simulink model "feedback_plant_with_simple_v2_PID"  (R2016a)
settings: Solver=FixedStepAuto  StartTime=0.0  StopTime=5580  MaxStep=0.1  RelTol=1e-3
undefined symbols (not defined in the file): sensors
libraries: slrtlib x10, simulink x3, xpcnilib x2
settings Model: ModifiedByFormat=The MathWorks Inc.  Creator=The MathWorks, Inc.  LastModifiedBy=The MathWorks Inc.
settings SolverCC: EnableConcurrentExecution=on
settings DataIOCC: LimitDataPoints=on  SaveFormat=Array
settings OptimizationCC: BlockReduction=off  DefaultParameterBehavior=Inlined  OptimizeBlockIOStorage=off  BufferReuse=off  GlobalBufferReuse=off  ExpressionFolding=off  ExpressionDepthLimit=2147483647  LocalBlockOutputs=off
settings DebuggingCC: UnderspecifiedInitializationDetection=Classic  MergeDetectMultiDrivingBlocksExec=none  SolverPrmCheckMsg=warning  FcnCallInpInsideContextMsg=EnableAllAsWarning  AllowSymbolicDim=off  StateNameClashWarn=warning
settings HardwareCC: ProdBitPerPointer=32  ProdLargestAtomicFloat=None  ProdWordSize=32  ProdLongLongMode=on  ProdHWDeviceType=Generic->32-bit x86 compatible
settings ModelReferenceCC: ModelReferenceNumInstancesAllowed=Single  ModelReferenceMinAlgLoopOccurrences=on  PropagateSignalLabelsOutOfModel=off
settings RTWCC: SystemTargetFile=slrt.tlc  TemplateMakefile=slrt_default_tmf  Description=Simulink Real-Time  RTWVerbose=off
settings ConfigComp: CovModelRefEnable=Off  CovSFcnEnable=off

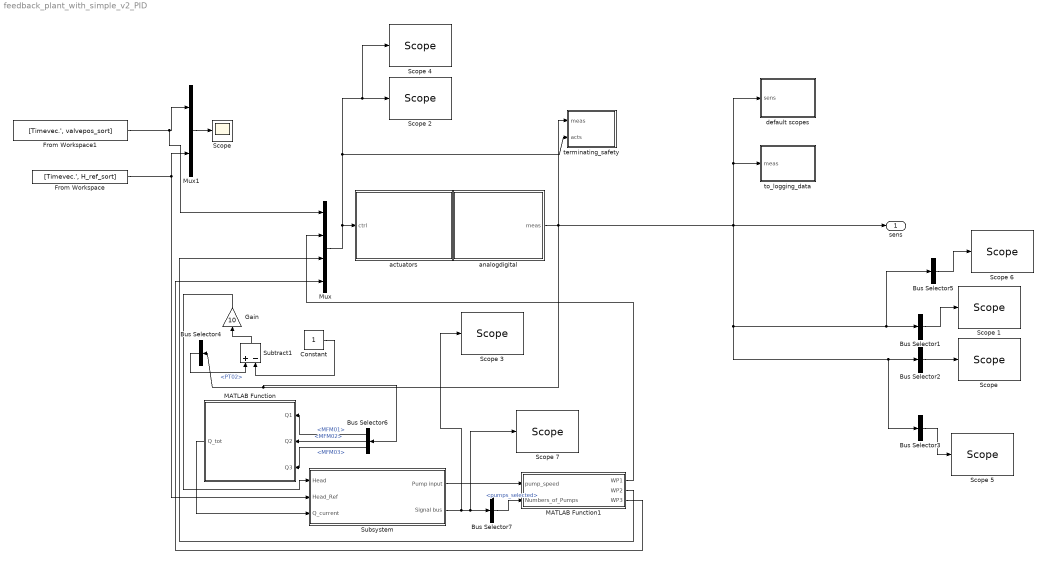
== system feedback_plant_with_simple_v2_PID ==
  Bus Selector1 : BusSelector  OutputSignals=CV01,DPT01,DPT02,DPT03,MFM01,MFM02,MFM03,PT02  OutputAsBus=on
  Bus Selector2 : BusSelector  OutputSignals=LMGV1,LMGV2,LMGV3,LMGC1,LMGC2,LMGC3,LMGP1,LMGP2,LMGP3  OutputAsBus=on
  Bus Selector3 : BusSelector  OutputSignals=WP01,WP02,WP03  OutputAsBus=on
  Bus Selector4 : BusSelector  OutputSignals=PT02
  Bus Selector5 : BusSelector  OutputSignals=PT02  OutputAsBus=on
  Bus Selector6 : BusSelector  OutputSignals=MFM01,MFM02,MFM03
  Bus Selector7 : BusSelector  OutputSignals=pumps_selected
  Constant : Constant
  From Workspace : FromWorkspace  VariableName=[Timevec.', H_ref_sort]  SampleTime=0  Interpolate=off  OutputAfterFinalValue=Holding final value
  From Workspace1 : FromWorkspace  VariableName=[Timevec.', valvepos_sort]  SampleTime=0  Interpolate=off  OutputAfterFinalValue=Holding final value
  Gain : Gain  Gain=10
  MATLAB Function : MATLAB Function  TreatAsAtomicUnit=on
  MATLAB Function1 : MATLAB Function  TreatAsAtomicUnit=on
  Mux : Mux
  Mux1 : Mux  Inputs=2
  Scope : Scope
  "Scope " : slrtlib/Displays and Logging/Scope   scopeno=9  scopetype=Target  autostart=on  viewmode=Numerical  formatstr='%15.6f'  grid=on  ylimits=[0,0]  nosamples=25  noprepostsamples=0  interleave=1  triggermode=FreeRun  triggersignal=1  trigsignalfromport=off  triggerlevel=0.0  triggerslope=Either  triggerscope=1  triggersample=0  filename=data.dat  mode=Lazy  writesize=512  autorestart=off  dynamicfilemode=off  maxwritefilesize=512*1024^2
  Scope 1 : slrtlib/Displays and Logging/Scope   scopeno=10  scopetype=Target  autostart=on  viewmode=Numerical  formatstr='%15.6f'  grid=on  ylimits=[0,0]  nosamples=25  noprepostsamples=0  interleave=1  triggermode=FreeRun  triggersignal=1  trigsignalfromport=off  triggerlevel=0.0  triggerslope=Either  triggerscope=1  triggersample=0  filename=data.dat  mode=Lazy  writesize=512  autorestart=off  dynamicfilemode=off  maxwritefilesize=512*1024^2
  Scope 2 : slrtlib/Displays and Logging/Scope   scopeno=2  scopetype=Host  autostart=on  viewmode=Graphical redraw  formatstr='%15.6f'  grid=on  ylimits=[0,0]  nosamples=250  noprepostsamples=0  interleave=1  triggermode=FreeRun  triggersignal=1  trigsignalfromport=off  triggerlevel=0.0  triggerslope=Either  triggerscope=1  triggersample=0  filename=data.dat  mode=Lazy  writesize=512  autorestart=off  dynamicfilemode=off  maxwritefilesize=512*1024^2
  Scope 3 : slrtlib/Displays and Logging/Scope   scopeno=3  scopetype=Host  autostart=on  viewmode=Graphical redraw  formatstr='%15.6f'  grid=on  ylimits=[0,0]  nosamples=250  noprepostsamples=0  interleave=1  triggermode=FreeRun  triggersignal=1  trigsignalfromport=off  triggerlevel=0.0  triggerslope=Either  triggerscope=1  triggersample=0  filename=data.dat  mode=Lazy  writesize=512  autorestart=off  dynamicfilemode=off  maxwritefilesize=512*1024^2
  Scope 4 : slrtlib/Displays and Logging/Scope   scopeno=8  scopetype=Target  autostart=on  viewmode=Numerical  formatstr='%15.6f'  grid=on  ylimits=[0,0]  nosamples=25  noprepostsamples=0  interleave=1  triggermode=FreeRun  triggersignal=1  trigsignalfromport=off  triggerlevel=0.0  triggerslope=Either  triggerscope=1  triggersample=0  filename=data.dat  mode=Lazy  writesize=512  autorestart=off  dynamicfilemode=off  maxwritefilesize=512*1024^2
  Scope 5 : slrtlib/Displays and Logging/Scope   scopeno=11  scopetype=Target  autostart=on  viewmode=Numerical  formatstr='%15.6f'  grid=on  ylimits=[0,0]  nosamples=25  noprepostsamples=0  interleave=1  triggermode=FreeRun  triggersignal=1  trigsignalfromport=off  triggerlevel=0.0  triggerslope=Either  triggerscope=1  triggersample=0  filename=data.dat  mode=Lazy  writesize=512  autorestart=off  dynamicfilemode=off  maxwritefilesize=512*1024^2
  Scope 6 : slrtlib/Displays and Logging/Scope   scopeno=4  scopetype=Target  autostart=on  viewmode=Graphical sliding  formatstr='%15.6f'  grid=on  ylimits=[0,0]  nosamples=100  noprepostsamples=0  interleave=1  triggermode=FreeRun  triggersignal=1  trigsignalfromport=off  triggerlevel=0.0  triggerslope=Either  triggerscope=1  triggersample=0  filename=data.dat  mode=Lazy  writesize=512  autorestart=off  dynamicfilemode=off  maxwritefilesize=512*1024^2
  Scope 7 : slrtlib/Displays and Logging/Scope   scopeno=6  scopetype=Target  autostart=on  viewmode=Numerical  formatstr='%15.6f'  grid=on  ylimits=[0,0]  nosamples=25  noprepostsamples=0  interleave=1  triggermode=FreeRun  triggersignal=1  trigsignalfromport=off  triggerlevel=0.0  triggerslope=Either  triggerscope=1  triggersample=0  filename=data.dat  mode=Lazy  writesize=512  autorestart=off  dynamicfilemode=off  maxwritefilesize=512*1024^2
  Subsystem : Subsystem
  Subtract1 : Sum  Inputs=+-
  actuators : Subsystem  mask{actuators_list={'CV03', 'CV05'}, subsystem=[3,1]}
      mask init:
      | %%Get analog channels
      | actuators = evalin('base','actuators');
      | 
      | subsystem = sprintf('[%d,%d]', subsystem(1), subsystem(2));
      | 
      | %actuators = actuators(strcmp(subsystem,{actuators.PCIslot}));
      | 
      | src_block = find_system(gcb, 'LookUnderMasks', 'on','Name', 'DA_sink');
      | maskObj = Simulink.Mask.get(src_block{1});
      | 
      | if(isempty(actuators))
      |    error('There are no analog outputs in the given card'); 
      | end
      | 
      | maskObj.Parameters(1,5).Value = subsystem;
      | maskObj.Parameters(1,1).Value = mat2str([actuators.Channel]+1);
      | Simulink.Block.eval(src_block{1});
      | 
      | %Find block
      | transform_blk = find_system(gcb, 'LookUnderMasks', 'on','Name', 'transform');
      | 
      | outputnames = {actuators.Name};
      | outputs = strjoin(outputnames,',');
      | 
      | sigcount = numel(outputnames);
      | sigstring = num2str(sigcount);
      | 
      | %Transform block
      | transform_blk = find_system(gcb, 'LookUnderMasks', 'on','Name', 'transform');
      | lines{1}=['function [' outputs ']  = fcn(u,gain,offset)'];
      | lines{2}='   y = u.*gain-offset;';
      | for i=1:numel(outputnames)
      |    %start at 4
      |    lines{2+i} = [ outputnames{i} ' = y(' num2str(i) ');'];
      | end
      | outputscript = strjoin(lines,'\n');
      | matlabfunctionfromstring(transform_blk{1}, outputscript);
      | Simulink.Block.eval(transform_blk{1});
      | 
      | %Delete lines
      | connections = find_system(gcb,'findall','on','LookUnderMasks', 'on','SearchDepth', 1,'type','line');
      | delete_line(connections);
      | 
      | for i=1:numel(outputnames)
      |    add_line(gcb,['transform/' num2str(i) ],['DA_sink/' num2str(i)],'autorouting','on');
      | end
      | 
      | %Transform block
      | add_line(gcb,'ctrl/1','transform/1','autorouting','on')
      | add_line(gcb,'gain/1','transform/2','autorouting','on')
      | add_line(gcb,'offset/1','transform/3','autorouting','on')
      | 
      | gain = [actuators.Gain]';
      | offset = [actuators.Offset]';
  analogdigital : Subsystem  mask{gain=[sensors.Gain], offset=[sensors.Offset]}
      mask init:
      | %%Get analog channels
      | sensors = evalin('base','sensors');
      | 
      | %subsystem = sprintf('[%d,%d]', subsystem(1), subsystem(2));
      | 
      | %analogin = sensors(strcmp(subsystem,{sensors.PCIslot})&(strcmp('VI|0-10V',{sensors.Type})|strcmp('VI|2-10V',{sensors.Type})|strcmp('CI|4-20mA',{sensors.Type})));
      | if ~isempty(sensors)
      | %    disp(['PCI slot ' subsystem ' loading']);
      | else
      |     error('There are no analog inputs in the given card'); 
      | end
      | 
      | 
      | %%Find source (ADC) block
      | src_block = find_system(gcb, 'LookUnderMasks', 'on','Name', 'src');
      | maskObj = Simulink.Mask.get(src_block{1});
      | 
      | %maskObj.Parameters(1,6).Value = subsystem;
      | maskObj.Parameters(1,1).Value = mat2str([sensors.Channel]+1);
      | Simulink.Block.eval(src_block{1});
      | 
      | %Find block
      | transform_blk = find_system(gcb, 'LookUnderMasks', 'on','Name', 'transform');
      | 
      | outputnames = {sensors.Name};
      | outputs = strjoin(outputnames,',');
      | 
      | sigcount = numel(outputnames);
      | sigstring = num2str(sigcount);
      | 
      | %Transform block
      | transform_blk = find_system(gcb, 'LookUnderMasks', 'on','Name', 'transform');
      | lines{1}=['function [' outputs ']  = fcn(u,gain,offset)'];
      | lines{2}='   y = u(:).*gain(:)-offset(:);';
      | for i=1:numel(outputnames)
      |    %start at 4
      |    lines{2+i} = [ outputnames{i} ' = y(' num2str(i) ');'];
      | end
      | outputscript = strjoin(lines,'\n');
      | matlabfunctionfromstring(transform_blk{1}, outputscript);
      | Simulink.Block.eval(transform_blk{1});
      | 
      | %Delete lines
      | connections = find_system(gcb,'findall','on','LookUnderMasks', 'on','SearchDepth', 1,'type','line');
      | delete_line(connections);
      | 
      | %Mux block
      | mux_blk = find_system(gcb, 'LookUnderMasks', 'on','Name', 'mux');
      | set_param(mux_blk{1},'Inputs', sigstring);
      | Simulink.Block.eval(mux_blk{1});
      | 
      | %Bus block
      | bus_blk = find_system(gcb, 'LookUnderMasks', 'on','Name', 'bus');
      | set_param(bus_blk{1},'Inputs', sigstring);
      | Simulink.Block.eval(bus_blk{1});
      | 
      | for i=1:numel(outputnames)
      |    add_line(gcb,['src/' num2str(i) ],['mux/' num2str(i)],'autorouting','on');
      |    add_line(gcb,['transform/' num2str(i) ],['bus/' num2str(i)],'autorouting','on');
      | end
      | 
      | %Lines to bus block
      | p = get_param(transform_blk, 'PortHandles');
      | l = get_param(p{1}.Outport,'Line');
      | 
      | for i=1:numel(outputnames)
      |    set_param(l{i},'Name',outputnames{i}) 
      | end
      | 
      | %Transform block
      | add_line(gcb,'mux/1','transform/1','autorouting','on')
      | add_line(gcb,'bus/1','meas/1','autorouting','on')
  default scopes : Subsystem
  terminating_safety : Subsystem
      mask init:
      | str1 = evalin('base', 'strjoin({sensors.Name},''/'')');
      | sensnames = uint8(str1);
  to_logging_data : Subsystem
  sens : Outport
  wires:
  Mux/1 -> actuators/1(ctrl), terminating_safety/2(acts), Scope 4/1, Scope 2/1
  analogdigital/1(meas) -> terminating_safety/1(meas), Bus Selector6/1, Bus Selector4/1, default scopes/1(sens), to_logging_data/1(meas), Bus Selector5/1, Bus Selector1/1, Bus Selector3/1, Bus Selector2/1, sens/1
  Bus Selector2/1 -> "Scope "/1
  Bus Selector1/1 -> Scope 1/1
  Mux1/1 -> Scope/1
  From Workspace1/1 -> Mux/1, Mux1/1
  From Workspace/1 -> Subsystem/2(Head_Ref), Mux1/2
  Bus Selector3/1 -> Scope 5/1
  Gain/1 -> Subsystem/1(Head)
  Bus Selector5/1 -> Scope 6/1
  Bus Selector6/2 -> MATLAB Function/2(Q2)  "<MFM02>"
  Bus Selector6/1 -> MATLAB Function/1(Q1)  "<MFM01>"
  Bus Selector6/3 -> MATLAB Function/3(Q3)  "<MFM03>"
  MATLAB Function/1(Q_tot) -> Subsystem/3(Q_current)
  Subsystem/1("Pump input ") -> MATLAB Function1/1(pump_speed)
  Subsystem/2(Signal bus) -> Scope 3/1, Scope 7/1, Bus Selector7/1
  MATLAB Function1/1(WP1) -> Mux/2
  MATLAB Function1/2(WP2) -> Mux/3
  MATLAB Function1/3(WP3) -> Mux/4
  Bus Selector4/1 -> Subtract1/1  "<PT02>"
  Subtract1/1 -> Gain/1
  Constant/1 -> Subtract1/2
  Bus Selector7/1 -> MATLAB Function1/2(Numbers_of_Pumps)  "<pumps_selected>"

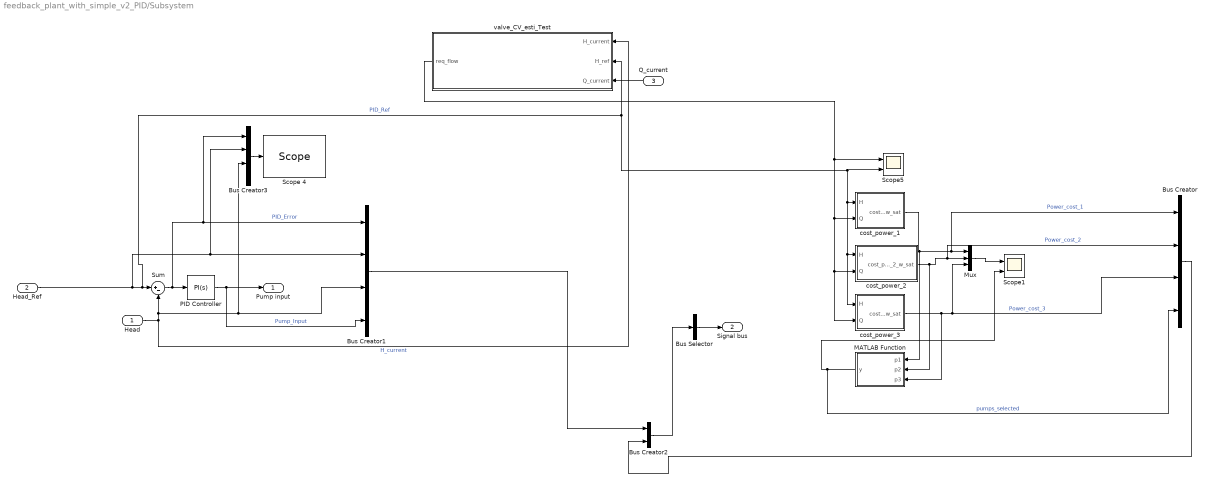
== system feedback_plant_with_simple_v2_PID/Subsystem ==
  Head : Inport
  Head_Ref : Inport  Port=2
  Q_current : Inport  Port=3
  Bus Creator : BusCreator  Inputs=4
  Bus Creator1 : BusCreator  Inputs=4
  Bus Creator2 : BusCreator  Inputs=2
  Bus Creator3 : BusCreator  Inputs=4
  Bus Selector : BusSelector  OutputSignals=signal1.PID_Error,signal1.PID_Ref,signal1.Pump_Input,signal2.Power_cost_1,signal2.Power_cost_2,signal2.Power_cost_3,signal2.pumps_selected,signal1.H_current  OutputAsBus=on
  MATLAB Function : MATLAB Function  TreatAsAtomicUnit=on
  Mux : Mux  Inputs=3
  PID Controller : simulink/Continuous/PID Controller  Controller=PI  TimeDomain=Continuous-time  SampleTime=-1  IntegratorMethod=Forward Euler  FilterMethod=Forward Euler  Form=Parallel  UseFilter=on  ControllerParametersSource=internal  P=0.03  I=0.04  D=0  N=100  InitialConditionSource=internal  InitialConditionForIntegrator=0  InitialConditionForFilter=0  ExternalReset=none  LimitOutput=on  UpperSaturationLimit=1  LowerSaturationLimit=0  LinearizeAsGain=on  AntiWindupMode=clamping  Kb=1  TrackingMode=off  Kt=1  PParamMin=[]  PParamMax=[]  IParamMin=[]  IParamMax=[]  DParamMin=[]  DParamMax=[]  NParamMin=[]  NParamMax=[]  KbParamMin=[]  KbParamMax=[]  KtParamMin=[]  KtParamMax=[]  POutMin=[]  POutMax=[]  IOutMin=[]  IOutMax=[]  DOutMin=[]  DOutMax=[]  NOutMin=[]  NOutMax=[]  KbOutMin=[]  KbOutMax=[]  KtOutMin=[]  KtOutMax=[]  IntegratorOutMin=[]  IntegratorOutMax=[]  FilterOutMin=[]  FilterOutMax=[]  SumOutMin=[]  SumOutMax=[]  SumI1OutMin=[]  SumI1OutMax=[]  SumI2OutMin=[]  SumI2OutMax=[]  SumI3OutMin=[]  SumI3OutMax=[]  SumDOutMin=[]  SumDOutMax=[]  SaturationOutMin=[]  SaturationOutMax=[]  IntegratorContinuousStateAttributes=''  IntegratorStateMustResolveToSignalObject=off  IntegratorRTWStateStorageClass=Auto  FilterContinuousStateAttributes=''  FilterStateMustResolveToSignalObject=off  FilterRTWStateStorageClass=Auto  DifferentiatorICPrevScaledInput=0  DifferentiatorOutMin=[]  DifferentiatorOutMax=[]
  Scope 4 : slrtlib/Displays and Logging/Scope   scopeno=5  scopetype=Target  autostart=on  viewmode=Numerical  formatstr='%15.6f'  grid=on  ylimits=[0,0]  nosamples=25  noprepostsamples=0  interleave=1  triggermode=FreeRun  triggersignal=1  trigsignalfromport=off  triggerlevel=0.0  triggerslope=Either  triggerscope=1  triggersample=0  filename=data.dat  mode=Lazy  writesize=512  autorestart=off  dynamicfilemode=off  maxwritefilesize=512*1024^2
  Scope1 : Scope  NumInputPorts=2
  Scope5 : Scope  NumInputPorts=2
  Sum : Sum  Inputs=|+-
  cost_power_1 : MATLAB Function  TreatAsAtomicUnit=on
  cost_power_2 : MATLAB Function  TreatAsAtomicUnit=on
  cost_power_3 : MATLAB Function  TreatAsAtomicUnit=on
  valve_CV_esti_Test : MATLAB Function  TreatAsAtomicUnit=on
  "Pump input " : Outport
  Signal bus : Outport  Port=2
  wires:
  cost_power_1/1(cost_power_1_w_sat) -> Bus Creator/1, Mux/1, MATLAB Function/1(p1)  "Power_cost_1"
  cost_power_2/1(cost_power_2_w_sat) -> Bus Creator/2, Mux/2, MATLAB Function/2(p2)  "Power_cost_2"
  cost_power_3/1(cost_power_3_w_sat) -> Bus Creator/3, Mux/3, MATLAB Function/3(p3)  "Power_cost_3"
  valve_CV_esti_Test/1(req_flow) -> Scope5/1, cost_power_1/2(Q), cost_power_2/2(Q), cost_power_3/2(Q)
  Head/1 -> Bus Creator3/3, Bus Creator1/3, Sum/2, valve_CV_esti_Test/1(H_current)  "H_current"
  Sum/1 -> PID Controller/1, Bus Creator3/1, Bus Creator1/1  "PID_Error"
  Head_Ref/1 -> Bus Creator3/2, Bus Creator1/2, valve_CV_esti_Test/2(H_ref), cost_power_1/1(H), cost_power_2/1(H), cost_power_3/1(H), Scope5/2, Sum/1  "PID_Ref"
  Q_current/1 -> valve_CV_esti_Test/3(Q_current)
  PID Controller/1 -> "Pump input "/1, Bus Creator1/4  "Pump_Input"
  Bus Creator/1 -> Bus Creator2/2
  MATLAB Function/1(y) -> Bus Creator/4, Scope1/2  "pumps_selected"
  Bus Creator1/1 -> Bus Creator2/1
  Bus Creator2/1 -> Bus Selector/1
  Mux/1 -> Scope1/1
  Bus Selector/1 -> Signal bus/1
  Bus Creator3/1 -> Scope 4/1

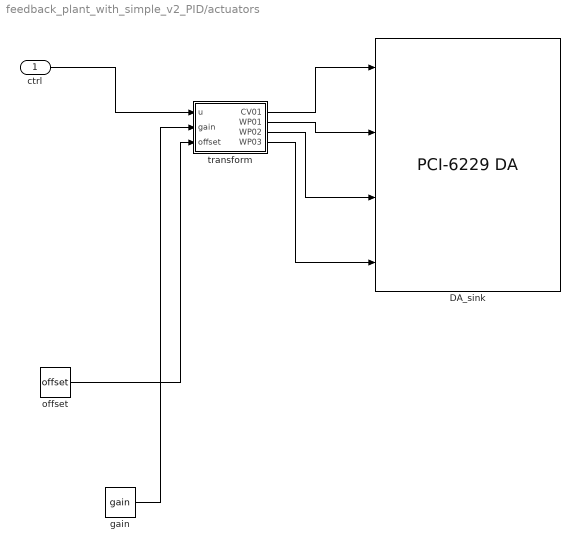
== system feedback_plant_with_simple_v2_PID/actuators ==
  ctrl : Inport
  DA_sink : xpcnilib/D//A/M Series/PCI-6229 DA  channel=[4 1 2 3]  reset=[1]  initValue=[0]  sampletime=0.01  slot=[3,1]
  gain : Constant  Value=gain
  offset : Constant  Value=offset
  transform : MATLAB Function  TreatAsAtomicUnit=on
  wires:
  transform/1(CV01) -> DA_sink/1
  transform/2(WP01) -> DA_sink/2
  transform/3(WP02) -> DA_sink/3
  transform/4(WP03) -> DA_sink/4
  ctrl/1 -> transform/1(u)
  gain/1 -> transform/2(gain)
  offset/1 -> transform/3(offset)

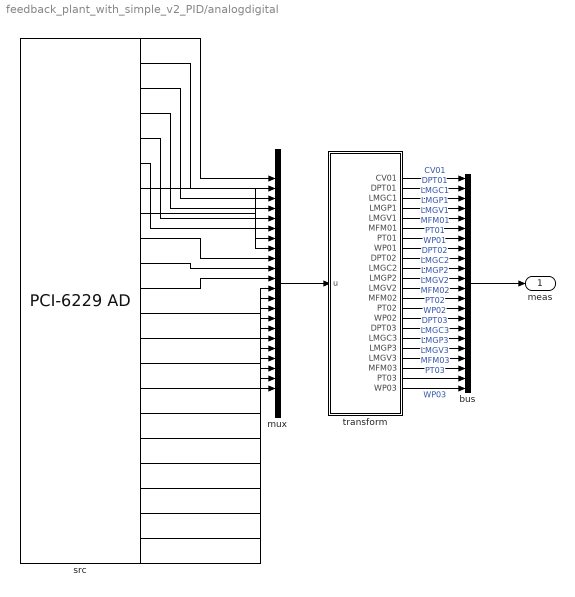
== system feedback_plant_with_simple_v2_PID/analogdigital ==
  bus : BusCreator  Inputs=22
  mux : Mux  Inputs=22
  src : xpcnilib/A//D/M Series/PCI-6229 AD  channel=[4 17 5 11 8 21 24 1 18 6 12 9 22 25 2 19 7 13 10 23 26 3]  range=[10]  coupling=[0]  scantime=5e-6  sampletime=0.01  slot=[3,1]
  transform : MATLAB Function  TreatAsAtomicUnit=on
  meas : Outport
  wires:
  src/1 -> mux/1
  transform/1(CV01) -> bus/1  "CV01"
  src/2 -> mux/2
  transform/2(DPT01) -> bus/2  "DPT01"
  src/3 -> mux/3
  transform/3(LMGC1) -> bus/3  "LMGC1"
  src/4 -> mux/4
  transform/4(LMGP1) -> bus/4  "LMGP1"
  src/5 -> mux/5
  transform/5(LMGV1) -> bus/5  "LMGV1"
  src/6 -> mux/6
  transform/6(MFM01) -> bus/6  "MFM01"
  src/7 -> mux/7
  transform/7(PT01) -> bus/7  "PT01"
  src/8 -> mux/8
  transform/8(WP01) -> bus/8  "WP01"
  src/9 -> mux/9
  transform/9(DPT02) -> bus/9  "DPT02"
  src/10 -> mux/10
  transform/10(LMGC2) -> bus/10  "LMGC2"
  src/11 -> mux/11
  transform/11(LMGP2) -> bus/11  "LMGP2"
  src/12 -> mux/12
  transform/12(LMGV2) -> bus/12  "LMGV2"
  src/13 -> mux/13
  transform/13(MFM02) -> bus/13  "MFM02"
  src/14 -> mux/14
  transform/14(PT02) -> bus/14  "PT02"
  src/15 -> mux/15
  transform/15(WP02) -> bus/15  "WP02"
  src/16 -> mux/16
  transform/16(DPT03) -> bus/16  "DPT03"
  src/17 -> mux/17
  transform/17(LMGC3) -> bus/17  "LMGC3"
  src/18 -> mux/18
  transform/18(LMGP3) -> bus/18  "LMGP3"
  src/19 -> mux/19
  transform/19(LMGV3) -> bus/19  "LMGV3"
  src/20 -> mux/20
  transform/20(MFM03) -> bus/20  "MFM03"
  src/21 -> mux/21
  transform/21(PT03) -> bus/21  "PT03"
  src/22 -> mux/22
  transform/22(WP03) -> bus/22  "WP03"
  mux/1 -> transform/1(u)
  bus/1 -> meas/1

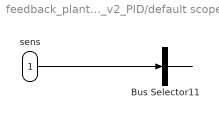
== system feedback_plant_with_simple_v2_PID/default scopes ==
  sens : Inport
  Bus Selector11 : BusSelector  OutputSignals=CV01,DPT01,LMGC1  OutputAsBus=on
  wires:
  sens/1 -> Bus Selector11/1
  Bus Selector11/1 -> ?

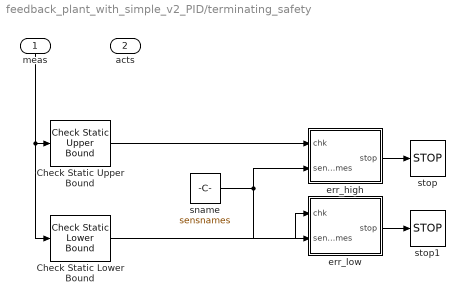
== system feedback_plant_with_simple_v2_PID/terminating_safety ==
  meas : Inport
  acts : Inport  Port=2
  Check Static Lower Bound : simulink/Model Verification/Check Static  Lower Bound  Description=[sensors.MinOp]-([sensors.MaxOp]-[sensors.MinOp])*0.05 <= u  min=[sensors.MinOp]-([sensors.MaxOp]-[sensors.MinOp])*0.05  min_included=on  enabled=on  stopWhenAssertionFail=off  export=on  icon=graphic
  Check Static Upper Bound : simulink/Model Verification/Check Static  Upper Bound  Description=u <= [sensors.MaxOp]+([sensors.MaxOp]-[sensors.MinOp])*0.05  max=[sensors.MaxOp]+([sensors.MaxOp]-[sensors.MinOp])*0.05  max_included=on  enabled=on  stopWhenAssertionFail=off  export=on  icon=graphic
  err_high : MATLAB Function  TreatAsAtomicUnit=on
  err_low : MATLAB Function  TreatAsAtomicUnit=on
  sname : Constant  Value=sensnames
  stop : Stop
  stop1 : Stop
  wires:
  Check Static Upper Bound/1 -> err_high/1(chk)
  Check Static Lower Bound/1 -> err_low/1(chk)
  sname/1 -> err_high/2(sensnames), err_low/2(sensnames)
  err_high/1(stop) -> stop/1
  err_low/1(stop) -> stop1/1
  meas/1 -> Check Static Lower Bound/1, Check Static Upper Bound/1

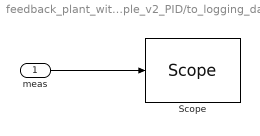
== system feedback_plant_with_simple_v2_PID/to_logging_data ==
  meas : Inport
  "Scope " : slrtlib/Displays and Logging/Scope   scopeno=1  scopetype=Host  autostart=on  viewmode=Graphical redraw  formatstr='%15.6f'  grid=on  ylimits=[0,0]  nosamples=250  noprepostsamples=0  interleave=1  triggermode=FreeRun  triggersignal=1  trigsignalfromport=off  triggerlevel=0.0  triggerslope=Either  triggerscope=1  triggersample=0  filename=data.dat  mode=Lazy  writesize=512  autorestart=off  dynamicfilemode=off  maxwritefilesize=512*1024^2
  wires:
  meas/1 -> "Scope "/1

== matlab function feedback_plant_with_simple_v2_PID/actuators/transform ==
  data: u input; CV01 output; gain input; offset input; WP01 output; WP02 output; WP03 output
function [CV01,WP01,WP02,WP03]  = fcn(u,gain,offset)
   y = u.*gain-offset;
CV01 = y(1);
WP01 = y(2);
WP02 = y(3);
WP03 = y(4);

== matlab function feedback_plant_with_simple_v2_PID/analogdigital/transform ==
  data: CV01 output size=1; u input; gain parameter; offset parameter; DPT01 output; LMGC1 output; LMGP1 output; LMGV1 output; MFM01 output; PT01 output; WP01 output; DPT02 output; LMGC2 output; LMGP2 output; LMGV2 output; MFM02 output; PT02 output; WP02 output; DPT03 output; LMGC3 output; LMGP3 output; LMGV3 output; MFM03 output; PT03 output; WP03 output
function [CV01,DPT01,LMGC1,LMGP1,LMGV1,MFM01,PT01,WP01,DPT02,LMGC2,LMGP2,LMGV2,MFM02,PT02,WP02,DPT03,LMGC3,LMGP3,LMGV3,MFM03,PT03,WP03]  = fcn(u,gain,offset)
   y = u(:).*gain(:)-offset(:);
CV01 = y(1);
DPT01 = y(2);
LMGC1 = y(3);
LMGP1 = y(4);
LMGV1 = y(5);
MFM01 = y(6);
PT01 = y(7);
WP01 = y(8);
DPT02 = y(9);
LMGC2 = y(10);
LMGP2 = y(11);
LMGV2 = y(12);
MFM02 = y(13);
PT02 = y(14);
WP02 = y(15);
DPT03 = y(16);
LMGC3 = y(17);
LMGP3 = y(18);
LMGV3 = y(19);
MFM03 = y(20);
PT03 = y(21);
WP03 = y(22);

== matlab function feedback_plant_with_simple_v2_PID/MATLAB Function ==
  data: Q1 input; Q_tot output; Q2 input; Q3 input
function Q_tot = fcn(Q1, Q2, Q3)

Q_tot = ((Q1 + Q2 + Q3) *60 * 60)/1000;

== matlab function feedback_plant_with_simple_v2_PID/MATLAB Function1 ==
  data: pump_speed input; WP1 output; Numbers_of_Pumps input; WP2 output; WP3 output
function [WP1, WP2, WP3] = fcn(pump_speed, Numbers_of_Pumps)
WP1 = 0;
WP2 = 0;
WP3 = 0;
if Numbers_of_Pumps == 1
    WP1 = pump_speed;
elseif Numbers_of_Pumps == 2
    WP1 = 1;
    WP2 = pump_speed;
elseif Numbers_of_Pumps == 3
    WP1 = 1;
    WP2 = 1;
    WP3 = pump_speed;
end

== matlab function feedback_plant_with_simple_v2_PID/Subsystem/MATLAB Function ==
  data: p1 input; y output; p2 input; p3 input
 function y = fcn(p1, p2, p3)
y = 1;
if p2 == 100000
    %2 pumps?
    y = 3;
elseif p1 == 50000
    y = 2;
    %3 pumps? 
end

== matlab function feedback_plant_with_simple_v2_PID/Subsystem/cost_power_1 ==
  data: cost_power_1_w_sat output; H input; Q input
function cost_power_1_w_sat = cost_power_1(H,Q)
%#codegen

%    This function was generated by the Symbolic Math Toolbox version 7.0.
%    22-Aug-2016 11:17:26

t2 = H.^5.314163576626763e-1;
t3 = t2.*4.673851686285024e2;
t4 = Q.^1.284992200316062;
t5 = t4.*9.427556616520734e1;
t13 = H.*Q.*3.590092811013802;
t6 = t3+t5-t13;
t7 = H.^1.157084314722127;
t8 = t7.*6.132915089183577;
t9 = Q.^2.682790628284203;
t10 = t9.*1.270953547543209;
t11 = H.*Q.*2.633327680950001;
t12 = t8+t10+t11;
cost_power_1_w_sat = double(((t6 <= 1.0e3) || (1.5e3 < t12)) || (3.5e3 <= t6)).*5.0e4+t12.*double(((1.0e3 < t6) && (t12 <= 1.5e3)) && (t6 < 3.5e3));

== matlab function feedback_plant_with_simple_v2_PID/Subsystem/cost_power_2 ==
  data: cost_power_2_w_sat output; H input; Q input
function cost_power_2_w_sat = cost_power_2(H,Q)
%#codegen

%    This function was generated by the Symbolic Math Toolbox version 7.0.
%    22-Aug-2016 11:17:26

t2 = Q.*(1.0./2.0);
t3 = t2.^1.284992200316062;
t4 = t3.*9.427556616520734e1;
t5 = H.^5.314163576626763e-1;
t6 = t5.*4.673851686285024e2;
t14 = H.*Q.*1.795046405506901;
t7 = t4+t6-t14;
t8 = H.^1.157084314722127;
t9 = t8.*6.132915089183577;
t10 = H.*Q.*1.316663840475001;
t11 = t2.^2.682790628284203;
t12 = t11.*1.270953547543209;
t13 = t9+t10+t12;
cost_power_2_w_sat = double(((t7 <= 1.0e3) || (1.5e3 < t13)) || (3.5e3 <= t7)).*1.0e5+t13.*double(((1.0e3 < t7) && (t13 <= 1.5e3)) && (t7 < 3.5e3)).*2.0;

== matlab function feedback_plant_with_simple_v2_PID/Subsystem/cost_power_3 ==
  data: cost_power_3_w_sat output; H input; Q input
function cost_power_3_w_sat = cost_power_3(H,Q)
%#codegen

%    This function was generated by the Symbolic Math Toolbox version 7.0.
%    22-Aug-2016 11:17:26

t2 = Q.*(1.0./3.0);
t3 = t2.^1.284992200316062;
t4 = t3.*9.427556616520734e1;
t5 = H.^5.314163576626763e-1;
t6 = t5.*4.673851686285024e2;
t14 = H.*Q.*1.196697603671267;
t7 = t4+t6-t14;
t8 = H.^1.157084314722127;
t9 = t8.*6.132915089183577;
t10 = H.*Q.*8.777758936500004e-1;
t11 = t2.^2.682790628284203;
t12 = t11.*1.270953547543209;
t13 = t9+t10+t12;
cost_power_3_w_sat = double(((t7 <= 1.0e3) || (1.5e3 < t13)) || (3.5e3 <= t7)).*1.5e5+t13.*double(((1.0e3 < t7) && (t13 <= 1.5e3)) && (t7 < 3.5e3)).*3.0;

== matlab function feedback_plant_with_simple_v2_PID/Subsystem/valve_CV_esti_Test ==
  data: H_current input; req_flow output; H_ref input; Q_current input
function req_flow = valve_CV_esti_Test(H_current,H_ref,Q_current)
%#codegen

%    This function was generated by the Symbolic Math Toolbox version 7.0.
%    22-Aug-2016 11:17:28

req_flow = 1.0./sqrt(H_current).*sqrt(H_ref).*Q_current;

== matlab function feedback_plant_with_simple_v2_PID/terminating_safety/err_high ==
  data: chk input; sensnames input uint8; stop output
function stop  = fcn(chk, sensnames)
%#codegen
%test = char(sensnames.');
test = sensnames.';
k = find(test == 47);
k = [0 k];
k = [k numel(test)];
stop = 0;
for i = 1:numel(chk)
    if chk(i) == 0
        str = char(test(k(i)+1:k(i+1)-1));
        Error = [str ': VALUE TOO HIGH ']
        coder.ceval('printf', ['%s' 10 0], Error);
        stop = stop+1;
    end
end

== matlab function feedback_plant_with_simple_v2_PID/terminating_safety/err_low ==
  data: chk input; sensnames input uint8; stop output
function stop  = fcn(chk, sensnames)
%#codegen
test = char(sensnames.');
k = strfind(test, '/');
k = [0 k];
k = [k numel(sensnames)];
stop = 0;
for i = 1:numel(chk)
    if chk(i) == 0
        str = char(test(k(i)+1:k(i+1)-1));
        Error = [str ': VALUE TOO LOW']
        coder.ceval('printf', ['%s' 10 0], Error);
        stop = stop+1;
    end
end
